simulink model "car"  (R2021a)
settings: Solver=VariableStepAuto  StartTime=0.0  StopTime=20  RelTol=1e-3
libraries: pid_lib x1
settings Model: Creator=Tony Pan  LastModifiedBy=Tony Pan

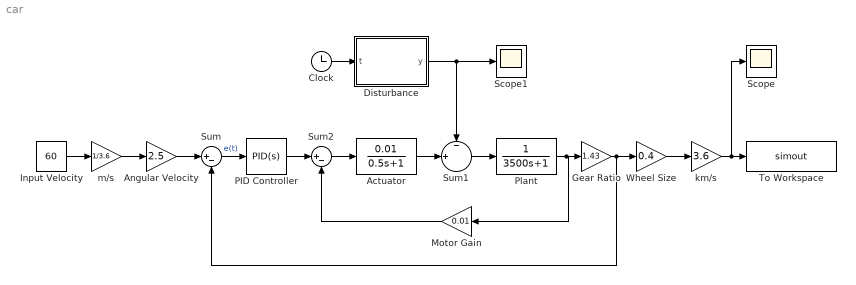
== system car ==
  Actuator : TransferFcn  Numerator=[0.01]  Denominator=[0.5 1]
  Angular Velocity : Gain  Gain=2.5
  Clock : Clock
  Disturbance : MATLAB Function  TreatAsAtomicUnit=on
  Gear Ratio : Gain  Gain=1.43
  Input Velocity : Constant  Value=60
  Motor Gain : Gain  Gain=0.01
  PID Controller : pid_lib/PID Controller  Controller=PID  Form=Parallel  TimeDomain=Continuous-time  UseExternalTs=off  SampleTime=-1  IntegratorMethod=Forward Euler  FilterMethod=Forward Euler  ControllerParametersSource=internal  P=2.4065e5  I=1.7909e4  D=3.8240e5  UseFilter=on  N=100  TunerSelectOption=Transfer Function Based (PID Tuner App)  InitialConditionSource=internal  InitialConditionForIntegrator=0  InitialConditionForFilter=0  DifferentiatorICPrevScaledInput=0  ExternalReset=none  TrackingMode=off  Kt=1  LimitOutput=off  SatLimitsSource=internal  UpperSaturationLimit=inf  LowerSaturationLimit=-inf  LinearizeAsGain=on  AntiWindupMode=none  Kb=1  POutMin=[]  POutMax=[]  IOutMin=[]  IOutMax=[]  DOutMin=[]  DOutMax=[]  NOutMin=[]  NOutMax=[]  SumOutMin=[]  SumOutMax=[]  SaturationOutMin=[]  SaturationOutMax=[]  PParamMin=[]  PParamMax=[]  IParamMin=[]  IParamMax=[]  DParamMin=[]  DParamMax=[]  NParamMin=[]  NParamMax=[]  KbParamMin=[]  KbParamMax=[]  KtParamMin=[]  KtParamMax=[]  KbOutMin=[]  KbOutMax=[]  KtOutMin=[]  KtOutMax=[]  IntegratorOutMin=[]  IntegratorOutMax=[]  FilterOutMin=[]  FilterOutMax=[]  SumI1OutMin=[]  SumI1OutMax=[]  SumI2OutMin=[]  SumI2OutMax=[]  SumI3OutMin=[]  SumI3OutMax=[]  SumI4OutMin=[]  SumI4OutMax=[]  SumDOutMin=[]  SumDOutMax=[]  DifferentiatorOutMin=[]  DifferentiatorOutMax=[]  FilterDiffOutCoefMin=[]  FilterDiffOutCoefMax=[]  ReciprocalOutMin=[]  ReciprocalOutMax=[]  SumDenOutMin=[]  SumDenOutMax=[]  SumNumOutMin=[]  SumNumOutMax=[]  DivideOutMin=[]  DivideOutMax=[]  UdiffTsProdOutMin=[]  UdiffTsProdOutMax=[]  NTsProdOutMin=[]  NTsProdOutMax=[]  UintegralTsProdOutMin=[]  UintegralTsProdOutMax=[]  UngainTsProdOutMin=[]  UngainTsProdOutMax=[]  IntegratorContinuousStateAttributes=''  IntegratorStateMustResolveToSignalObject=off  IntegratorRTWStateStorageClass=Auto  FilterContinuousStateAttributes=''  FilterStateMustResolveToSignalObject=off  FilterRTWStateStorageClass=Auto  ParallelPVariant=InternalParameters  IdealPVariant=Disabled  IVariant=InternalParameters  DVariant=InternalParameters  IntegratorVariant=Continuous  SatVariant=Disabled  AWVariant=Passthrough  PCopyVariant=Disabled  TRVariant=Disabled  FdbkBlocksVariant=Forward  IdealPFdbkVariant=Disabled  SatFdbkVariant=Disabled  DerivativeFilterVariant=ContFilter  NVariant=InternalParameters  NCopyVariant=Disabled  FilterICVariant=InternalICsFilter  IntegratorICVariant=InternalICs  ExternalResetVariant=Disabled  TRSumVariant=Passthrough  SumFdbkVariant=Disabled  SumVariant=Sum_PID  TsampFilterVariant=InternalTs  TsampNgainVariant=Passthrough  TsampIntegralVariant=Passthrough  ExternalSaturationOutDataTypeStr=Inherit: Same as second input
  Plant : TransferFcn  Denominator=[3500 1]
  Scope : Scope
  Scope1 : Scope
  Sum : Sum  Inputs=|+-
  Sum1 : Sum  Inputs=-|+||
  Sum2 : Sum  Inputs=|+-
  To Workspace : ToWorkspace  VariableName=simout  SaveFormat=Timeseries  SampleTime=-1
  Wheel Size : Gain  Gain=0.4
  km/s : Gain  Gain=3.6
  m/s : Gain  Gain=1/3.6
  wires:
  Sum/1 -> PID Controller/1  "e(t)"
  Plant/1 -> Motor Gain/1, Gear Ratio/1
  Actuator/1 -> Sum1/2
  Sum1/1 -> Plant/1
  Disturbance/1(y) -> Scope1/1, Sum1/1
  Clock/1 -> Disturbance/1(t)
  Sum2/1 -> Actuator/1
  PID Controller/1 -> Sum2/1
  Motor Gain/1 -> Sum2/2
  Gear Ratio/1 -> Sum/2, Wheel Size/1
  Angular Velocity/1 -> Sum/1
  Wheel Size/1 -> km/s/1
  km/s/1 -> Scope/1, To Workspace/1
  Input Velocity/1 -> m/s/1
  m/s/1 -> Angular Velocity/1

== matlab function car/Disturbance ==
  settings: updateMethod=DISCRETE
  data: t input; y output
function y = fcn(t)
    if mod(t, 30) < 10
        y = randi(5000) * sin(2 * t);
    elseif mod(t, 30) < 20
        y = randi(10000) * sin(2 * t);
    else
        y = randi(15000) * sin(2 * t);
    end
end
